simulink model "TurnLights_Model"  (R2025b)
settings: Solver=FixedStepAuto  StartTime=0.0  StopTime=4  RelTol=1e-3
settings Model: Creator=Sai Krishna  LastModifiedBy=Sai Krishna
settings DataIOCC: LoadExternalInput=on  DSMLogging=off  ReturnWorkspaceOutputs=off  LoggingToFile=on
settings OptimizationCC: DefaultParameterBehavior=Inlined  EnhancedBackFolding=on  PassReuseOutputArgsAs=Individual arguments  ZeroExternalMemoryAtStartup=off  ZeroInternalMemoryAtStartup=off  OptimizeBlockOrder=speed  DifferentSizesBufferReuse=on  OptimizationCustomize=off  EfficientTunableParamExpr=on
settings DebuggingCC: ParameterTunabilityLossMsg=error  BusObjectLabelMismatch=error
settings SFSimCC: MATLABDynamicMemAlloc=off
settings RTWCC: SystemTargetFile=ert.tlc  TemplateMakefile=ert_default_tmf  Description=Embedded Coder
settings CodeAppCC: ForceParamTrailComments=on  IgnoreCustomStorageClasses=off  OperatorAnnotations=on  SimulinkDataObjDesc=on  SFDataObjDesc=on  InsertBlockDesc=on
settings ERTTargetCC: ERTCustomFileTemplate=example_file_process.tlc  TargetLangStandard=C99 (ISO)  GenerateSampleERTMain=on

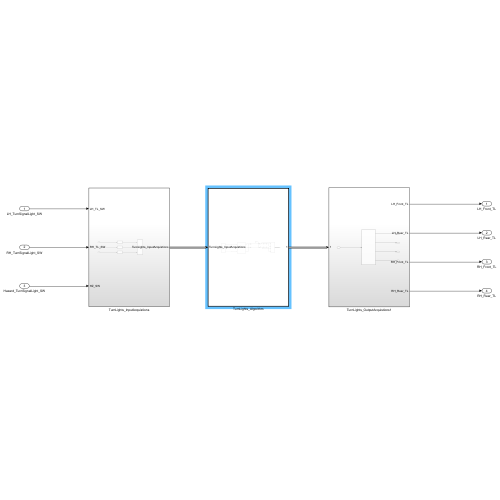
[thumbnail: Simulink's stored preview of the top-level diagram]
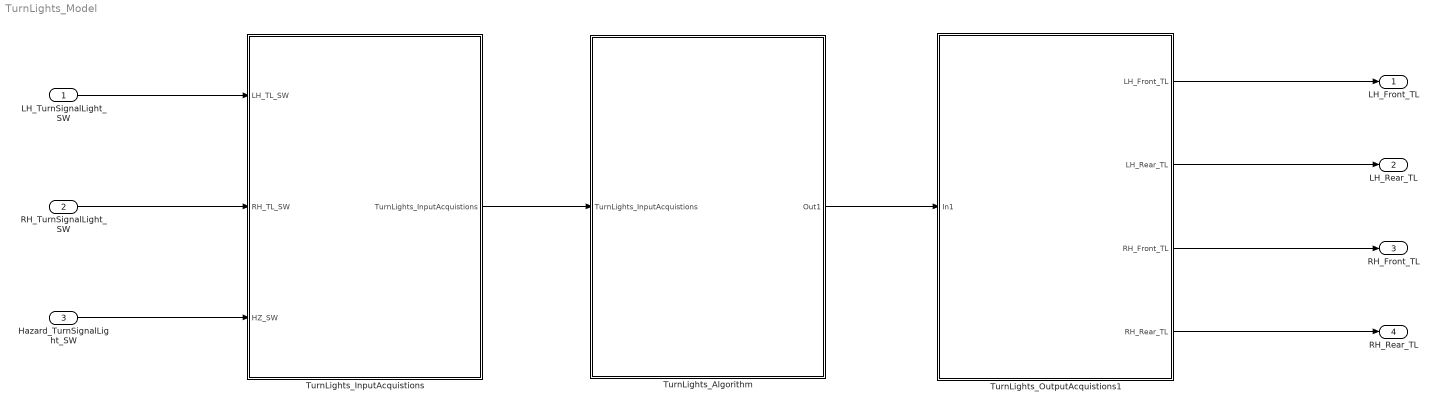
== system TurnLights_Model ==
  LH_TurnSignalLight_SW : Inport
  RH_TurnSignalLight_SW : Inport  Port=2
  Hazard_TurnSignalLight_SW : Inport  Port=3
  TurnLights_Algorithm : Subsystem  TreatAsAtomicUnit=on
  TurnLights_InputAcquistions : Subsystem
  TurnLights_OutputAcquistions1 : Subsystem
  LH_Front_TL : Outport
  LH_Rear_TL : Outport  Port=2
  RH_Front_TL : Outport  Port=3
  RH_Rear_TL : Outport  Port=4
  wires:
  LH_TurnSignalLight_SW/1 -> TurnLights_InputAcquistions/1(LH_TL_SW)
  RH_TurnSignalLight_SW/1 -> TurnLights_InputAcquistions/2(RH_TL_SW)
  Hazard_TurnSignalLight_SW/1 -> TurnLights_InputAcquistions/3(HZ_SW)
  TurnLights_InputAcquistions/1(TurnLights_InputAcquistions) -> TurnLights_Algorithm/1(TurnLights_InputAcquistions)
  TurnLights_Algorithm/1(Out1) -> TurnLights_OutputAcquistions1/1(In1)
  TurnLights_OutputAcquistions1/1(LH_Front_TL) -> LH_Front_TL/1
  TurnLights_OutputAcquistions1/2(LH_Rear_TL) -> LH_Rear_TL/1
  TurnLights_OutputAcquistions1/3(RH_Front_TL) -> RH_Front_TL/1
  TurnLights_OutputAcquistions1/4(RH_Rear_TL) -> RH_Rear_TL/1

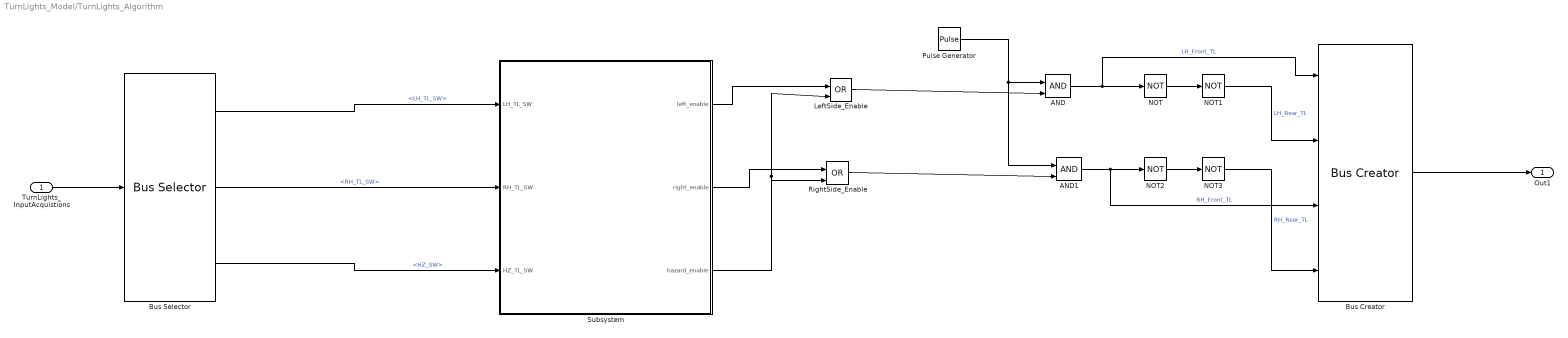
== system TurnLights_Model/TurnLights_Algorithm ==
  TurnLights_InputAcquistions : Inport
  AND : Logic  IconShape=distinctive  AllPortsSameDT=off  OutDataTypeStr=boolean
  AND1 : Logic  IconShape=distinctive  AllPortsSameDT=off  OutDataTypeStr=boolean
  Bus Creator : BusCreator  Inputs=4  OutDataTypeStr=Bus: TurnLight_OutputBus
      settings: InheritFromInputs=off
  Bus Selector : BusSelector  OutputSignals=LH_TL_SW,RH_TL_SW,HZ_SW
  LeftSide_Enable : Logic  Operator=OR  IconShape=distinctive  AllPortsSameDT=off  OutDataTypeStr=boolean
  NOT{,1..3} (4 alike) : Logic  Operator=NOT  IconShape=distinctive  AllPortsSameDT=off  OutDataTypeStr=boolean
  Pulse Generator : DiscretePulseGenerator  PulseType=Time based  Period=1  PulseWidth=50
  RightSide_Enable : Logic  Operator=OR  IconShape=distinctive  AllPortsSameDT=off  OutDataTypeStr=boolean
  Subsystem : Subsystem
  Out1 : Outport  OutDataTypeStr=Bus: TurnLight_OutputBus
  wires:
  TurnLights_InputAcquistions/1 -> Bus Selector/1
  RightSide_Enable/1 -> AND1/2
  LeftSide_Enable/1 -> AND/2
  Pulse Generator/1 -> AND1/1, AND/1
  Bus Creator/1 -> Out1/1
  Bus Selector/1 -> Subsystem/1(LH_TL_SW)  "<LH_TL_SW>"
  Bus Selector/2 -> Subsystem/2(RH_TL_SW)  "<RH_TL_SW>"
  Bus Selector/3 -> Subsystem/3(HZ_TL_SW)  "<HZ_SW>"
  Subsystem/1(left_enable) -> LeftSide_Enable/1
  Subsystem/2(right_enable) -> RightSide_Enable/1
  Subsystem/3(hazard_enable) -> RightSide_Enable/2, LeftSide_Enable/2
  AND/1 -> Bus Creator/1, NOT/1  "LH_Front_TL"
  NOT/1 -> NOT1/1
  NOT1/1 -> Bus Creator/2  "LH_Rear_TL"
  AND1/1 -> Bus Creator/3, NOT2/1  "RH_Front_TL"
  NOT2/1 -> NOT3/1
  NOT3/1 -> Bus Creator/4  "RH_Rear_TL"

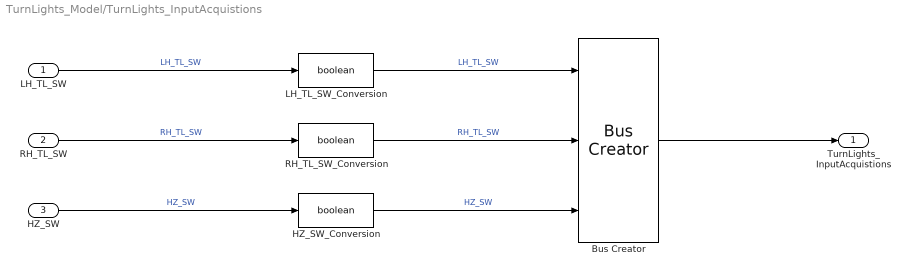
== system TurnLights_Model/TurnLights_InputAcquistions ==
  LH_TL_SW : Inport  OutDataTypeStr=boolean
  RH_TL_SW : Inport  Port=2  OutDataTypeStr=boolean
  HZ_SW : Inport  Port=3  OutDataTypeStr=boolean
  Bus Creator : BusCreator  Inputs=3  OutDataTypeStr=Bus: TurnLight_InputBus
      settings: InheritFromInputs=off
  HZ_SW_Conversion : DataTypeConversion  OutDataTypeStr=boolean  SaturateOnIntegerOverflow=off  RndMeth=Floor
  LH_TL_SW_Conversion : DataTypeConversion  OutDataTypeStr=boolean  SaturateOnIntegerOverflow=off  RndMeth=Floor
  RH_TL_SW_Conversion : DataTypeConversion  OutDataTypeStr=boolean  SaturateOnIntegerOverflow=off  RndMeth=Floor
  TurnLights_InputAcquistions : Outport  OutDataTypeStr=Bus: TurnLight_InputBus
  wires:
  LH_TL_SW/1 -> LH_TL_SW_Conversion/1  "LH_TL_SW"
  RH_TL_SW/1 -> RH_TL_SW_Conversion/1  "RH_TL_SW"
  Bus Creator/1 -> TurnLights_InputAcquistions/1
  RH_TL_SW_Conversion/1 -> Bus Creator/2  "RH_TL_SW"
  HZ_SW_Conversion/1 -> Bus Creator/3  "HZ_SW"
  HZ_SW/1 -> HZ_SW_Conversion/1  "HZ_SW"
  LH_TL_SW_Conversion/1 -> Bus Creator/1  "LH_TL_SW"

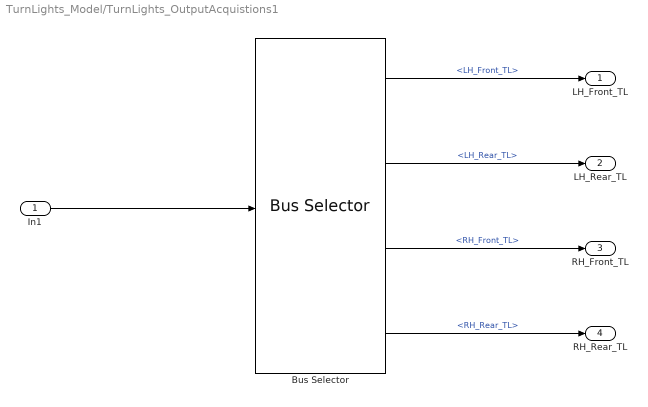
== system TurnLights_Model/TurnLights_OutputAcquistions1 ==
  In1 : Inport  OutDataTypeStr=Bus: TurnLight_OutputBus
  Bus Selector : BusSelector  OutputSignals=LH_Front_TL,LH_Rear_TL,RH_Front_TL,RH_Rear_TL
  LH_Front_TL : Outport
  LH_Rear_TL : Outport  Port=2
  RH_Front_TL : Outport  Port=3
  RH_Rear_TL : Outport  Port=4
  wires:
  Bus Selector/1 -> LH_Front_TL/1  "<LH_Front_TL>"
  Bus Selector/2 -> LH_Rear_TL/1  "<LH_Rear_TL>"
  Bus Selector/3 -> RH_Front_TL/1  "<RH_Front_TL>"
  Bus Selector/4 -> RH_Rear_TL/1  "<RH_Rear_TL>"
  In1/1 -> Bus Selector/1

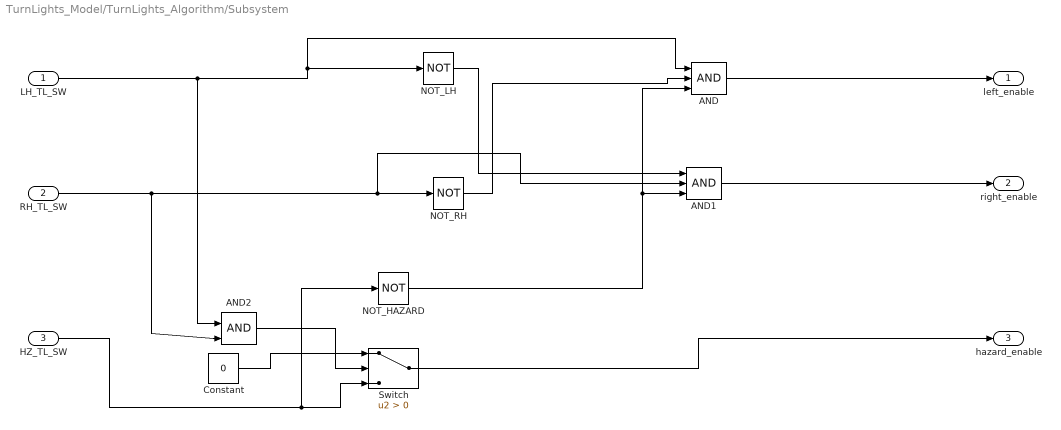
== system TurnLights_Model/TurnLights_Algorithm/Subsystem ==
  LH_TL_SW : Inport
  RH_TL_SW : Inport  Port=2
  HZ_TL_SW : Inport  Port=3
  AND : Logic  Inputs=3  IconShape=distinctive  AllPortsSameDT=off  OutDataTypeStr=boolean
  AND1 : Logic  Inputs=3  IconShape=distinctive  AllPortsSameDT=off  OutDataTypeStr=boolean
  AND2 : Logic  IconShape=distinctive  AllPortsSameDT=off  OutDataTypeStr=boolean
  Constant : Constant  Value=0  OutDataTypeStr=boolean
  NOT_HAZARD : Logic  Operator=NOT  AllPortsSameDT=off  OutDataTypeStr=boolean
  NOT_LH : Logic  Operator=NOT  AllPortsSameDT=off  OutDataTypeStr=boolean
  NOT_RH : Logic  Operator=NOT  AllPortsSameDT=off  OutDataTypeStr=boolean
  Switch : Switch  Criteria=u2 > Threshold  OutDataTypeStr=boolean  SaturateOnIntegerOverflow=off  InputSameDT=off
  left_enable : Outport
  right_enable : Outport  Port=2
  hazard_enable : Outport  Port=3
  wires:
  AND1/1 -> right_enable/1
  AND/1 -> left_enable/1
  LH_TL_SW/1 -> AND2/1, AND/1, NOT_LH/1
  RH_TL_SW/1 -> AND2/2, AND1/2, NOT_RH/1
  NOT_LH/1 -> AND1/1
  NOT_HAZARD/1 -> AND/3, AND1/3
  NOT_RH/1 -> AND/2
  AND2/1 -> Switch/2
  HZ_TL_SW/1 -> NOT_HAZARD/1, Switch/3
  Switch/1 -> hazard_enable/1
  Constant/1 -> Switch/1
